simulink model "MotorMitSchwungmasseONLY"  (R2023b)
settings: Solver=VariableStepAuto  StartTime=0.0  StopTime=10.0  RelTol=1e-3
libraries: Plants x1
settings Model: Creator=Alex  LastModifiedBy=Alex

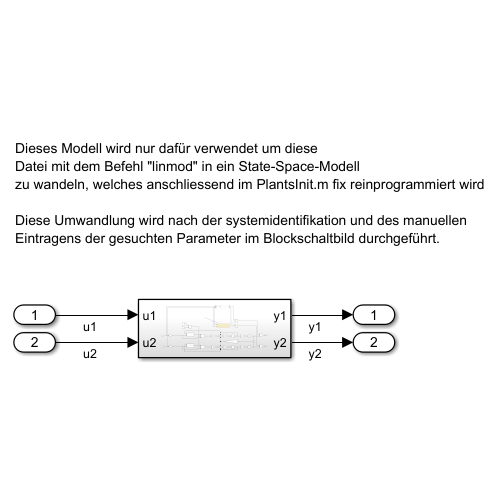
[thumbnail: Simulink's stored preview of the top-level diagram]
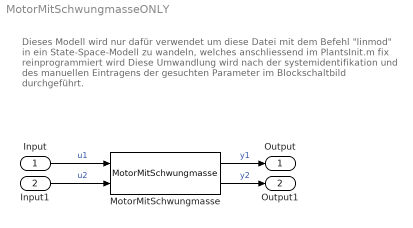
== system MotorMitSchwungmasseONLY ==
  note: Dieses Modell wird nur dafür verwendet um diese
      | Datei mit dem Befehl "linmod" in ein State-Space-Modell
      | zu wandeln, welches anschliessend im PlantsInit.m fix reinprogrammiert wird
      |
      | Diese Umwandlung wird nach der systemidentifikation und des manuellen
      | Eintragens der gesuchten Parameter im Blockschaltbild durchgeführt.
  Input : Inport
  Input1 : Inport  Port=2
  MotorMitSchwungmasse : Plants/MotorMitSchwungmasse  SystemSampleTime=-1  VariantActivationTime=update diagram  AllowFlexibleInterface=on  Latency=0  AutoFrameSizeCalculation=off
  Output : Outport
  Output1 : Outport  Port=2
  wires:
  Input/1 -> MotorMitSchwungmasse/1  "u1"
  Input1/1 -> MotorMitSchwungmasse/2  "u2"
  MotorMitSchwungmasse/1 -> Output/1  "y1"
  MotorMitSchwungmasse/2 -> Output1/1  "y2"
